simulink model "three_pole_pi_final"  (R2025b)
settings: Solver=VariableStepAuto  StartTime=0.0  StopTime=30  RelTol=1e-3
model workspace (MAT data in the model file):
  Ki = 7143
  Kp = 1546
  alpha = 17.4520069808
  beta = 0.0026
  l_eff = 0.4992
  omega_n = 4.4308
settings Model: Creator=clee1  LastModifiedBy=kyue
settings SolverCC: AlgebraicLoopSolver=TrustRegion
settings DebuggingCC: UnconnectedInputMsg=warning  UnconnectedOutputMsg=warning  UnconnectedLineMsg=warning
settings ModelReferenceCC: EnableRefExpFcnMdlSchedulingChecks=on
settings RTWCC: GPUComputeCapability=3.5

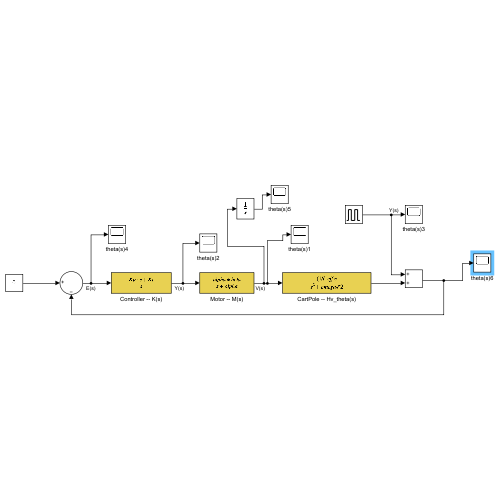
[thumbnail: Simulink's stored preview of the top-level diagram]
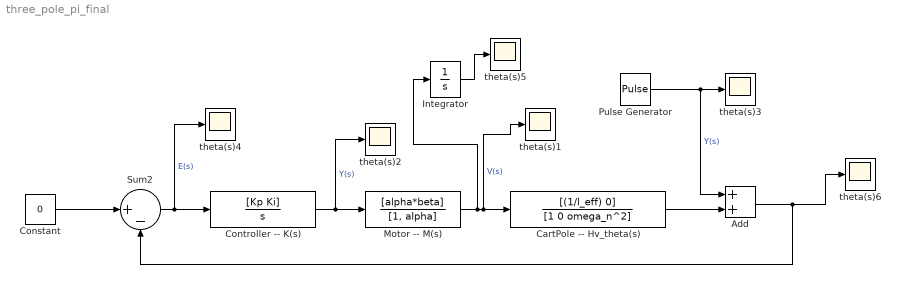
== system three_pole_pi_final ==
  Add : Sum
  "CartPole -- Hv_theta(s)" : TransferFcn  Numerator=[(1/l_eff) 0]  Denominator=[1 0 omega_n^2]  ContinuousStateAttributes="\"Controller\""
  Constant : Constant  Value=0
  "Controller -- K(s)" : TransferFcn  Numerator=[Kp Ki]  Denominator=[1 0]  ContinuousStateAttributes="\"Controller\""
  Integrator : Integrator
  "Motor -- M(s)" : TransferFcn  Numerator=[alpha*beta]  Denominator=[1, alpha]  ContinuousStateAttributes="\"Controller\""
  Pulse Generator : DiscretePulseGenerator  PulseType=Time based  Amplitude=.3  Period=7  PulseWidth=.1
  Sum2 : Sum  Inputs=|+-
  theta(s){1..6} (6 alike) : Scope
      theta(s)1 settings: ActiveDisplayYMinimum=-0.28036836099875995  ActiveDisplayYMaximum=0.075536987568240316
      theta(s)2 settings: ActiveDisplayYMinimum=-207123.87141520879  ActiveDisplayYMaximum=91376.996775463092  DataLoggingVariableName=ScopeData2
      theta(s)3 settings: ActiveDisplayYMinimum=-3.1697328457131824  ActiveDisplayYMaximum=2.5139612707542889  DataLoggingVariableName=ScopeData3
      theta(s)4 settings: ActiveDisplayYMinimum=-1  ActiveDisplayYMaximum=1  DataLoggingVariableName=ScopeData4
      theta(s)5 settings: ActiveDisplayYMinimum=0.18940750154394226  ActiveDisplayYMaximum=0.381027525934147  DataLoggingVariableName=ScopeData5
      theta(s)6 settings: ActiveDisplayYMinimum=-0.078958957250802708  ActiveDisplayYMaximum=0.40569836455782471
  wires:
  Sum2/1 -> theta(s)4/1, "Controller -- K(s)"/1  "E(s)"
  "Controller -- K(s)"/1 -> theta(s)2/1, "Motor -- M(s)"/1  "Y(s)"
  "Motor -- M(s)"/1 -> Integrator/1, theta(s)1/1, "CartPole -- Hv_theta(s)"/1  "V(s)"
  "CartPole -- Hv_theta(s)"/1 -> Add/2
  Constant/1 -> Sum2/1
  Add/1 -> Sum2/2, theta(s)6/1
  Pulse Generator/1 -> Add/1, theta(s)3/1  "Y(s)"
  Integrator/1 -> theta(s)5/1
